simulink model "gm_testing"  (R2023a)
settings: Solver=VariableStepAuto  StartTime=0.0  StopTime=inf  RelTol=1e-3
libraries: commdigbbndpm3 x1, commrandsrc3 x1, simulink x1
settings Model: Creator=acer  LastModifiedBy=acer
settings OptimizationCC: BlockReduction=off  ConditionallyExecuteInputs=off
settings DebuggingCC: InheritedTsInSrcMsg=none

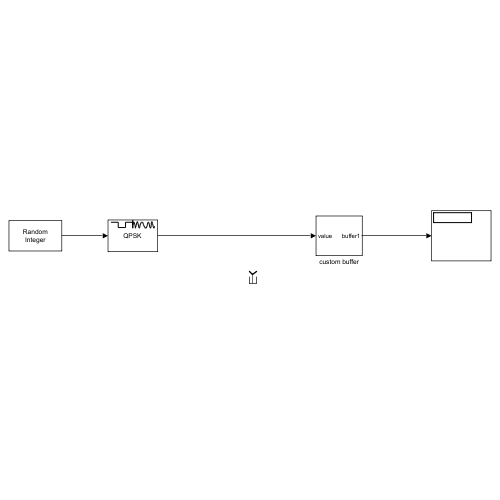
[thumbnail: Simulink's stored preview of the top-level diagram]
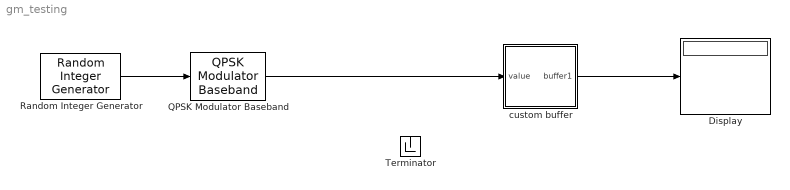
== system gm_testing ==
  Display : Display
  QPSK Modulator Baseband : commdigbbndpm3/QPSK Modulator Baseband  InType=Integer  Enc=Gray  Ph=pi/4  outDtype=Fixed-point  outWordLen=16  outUDDataType=sfix(16)  outFracLenMode=Best precision  outFracLen=15  outDataTypeStr=fixdt(1,16)  outLastDataTypeStr=fixdt(1,16)
      settings: LibrarySourceBlock=|
      | commhdldigbbndpm/QPSK
      | Modulator
      | Baseband
  Random Integer Generator : commrandsrc3/Random Integer Generator  SetSize=4  SeedSource=Auto  Seed=0  SampleTime=1  SamplesPerFrame=1  OutputDataType=uint8  SimulateUsing=Interpreted execution
  Terminator : Terminator
  custom buffer : Subsystem
  wires:
  QPSK Modulator Baseband/1 -> custom buffer/1(value)
  Random Integer Generator/1 -> QPSK Modulator Baseband/1
  custom buffer/1(buffer1) -> Display/1

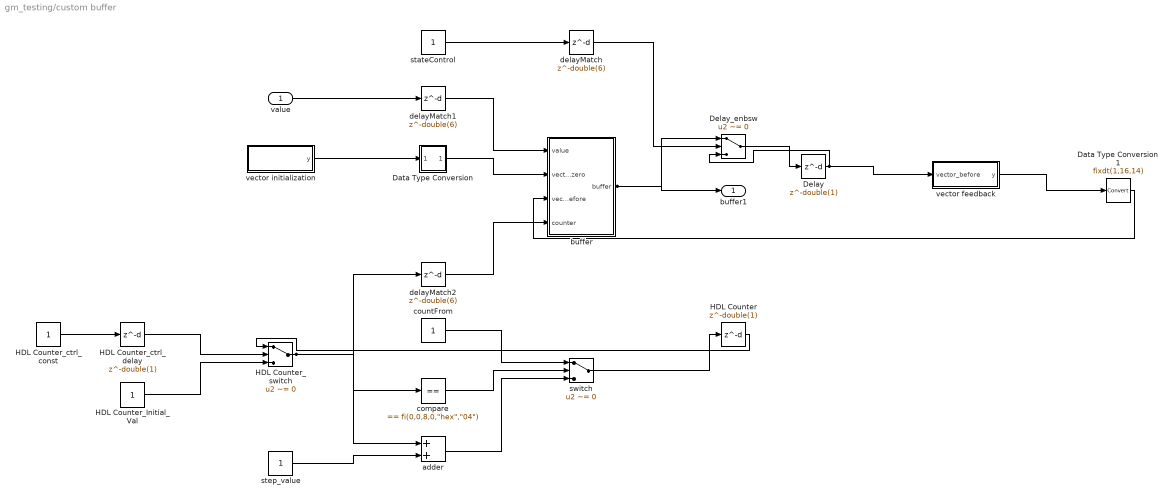
== system gm_testing/custom buffer ==
  value : Inport  OutDataTypeStr=fixdt(1, 16, 15)  PortDimensions=1  SampleTime=1
      settings: SignalType=complex
  Data Type Conversion : Subsystem
      mask Display: disp('NFP\nconv');
  Data Type Conversion1 : DataTypeConversion  OutDataTypeStr=fixdt(1,16,14)
  Delay : Delay  DelayLength=double(1)  InitialCondition=0  SampleTime=1
  Delay_enbsw : Switch  Criteria=u2 ~= 0  Threshold=double(0)  OutDataTypeStr=fixdt(1, 16, 14)  SampleTime=1  SaturateOnIntegerOverflow=off  InputSameDT=off
  HDL Counter : Delay  DelayLength=double(1)  InitialCondition=0  SampleTime=1
  HDL Counter_Initial_Val : Constant  OutDataTypeStr=uint8  SampleTime=1
  HDL Counter_ctrl_const : Constant  OutDataTypeStr=boolean  SampleTime=1
  HDL Counter_ctrl_delay : Delay  DelayLength=double(1)  InitialCondition=0  SampleTime=1
  HDL Counter_switch : Switch  Criteria=u2 ~= 0  Threshold=double(0)  OutDataTypeStr=uint8  SampleTime=1  SaturateOnIntegerOverflow=off  InputSameDT=off
  adder : Sum  AccumDataTypeStr=uint8  OutDataTypeStr=uint8  SampleTime=1
  buffer : Subsystem
  compare : simulink/Logic and Bit Operations/Compare To Constant  relop===  const="fi(0,0,8,0,\"hex\",\"04\")"  OutDataTypeStr=boolean
  countFrom : Constant  VectorParams1D=off  OutDataTypeStr=uint8  SampleTime=1
  delayMatch : Delay  DelayLength=double(6)  InitialCondition=0  SampleTime=1
  delayMatch1 : Delay  DelayLength=double(6)  InitialCondition=0  SampleTime=1
  delayMatch2 : Delay  DelayLength=double(6)  InitialCondition=0  SampleTime=1
  stateControl : Constant  OutDataTypeStr=boolean  SampleTime=1
  step_value : Constant  VectorParams1D=off  OutDataTypeStr=uint8  SampleTime=1
  switch : Switch  Criteria=u2 ~= 0  Threshold=double(0)  OutDataTypeStr=uint8  SampleTime=1  SaturateOnIntegerOverflow=off  InputSameDT=off
  vector feedback : Subsystem
  vector initialization : Subsystem
  buffer1 : Outport  SampleTime=1
  wires:
  delayMatch1/1 -> buffer/1(value)
  delayMatch2/1 -> buffer/4(counter)
  vector initialization/1(y) -> Data Type Conversion/1(In1)
  HDL Counter_switch/1 -> delayMatch2/1, compare/1, adder/1
  step_value/1 -> adder/2
  countFrom/1 -> switch/1
  HDL Counter_Initial_Val/1 -> HDL Counter_switch/3
  HDL Counter_ctrl_const/1 -> HDL Counter_ctrl_delay/1
  HDL Counter_ctrl_delay/1 -> HDL Counter_switch/2
  Data Type Conversion/1(Out1) -> buffer/2(vector_zero)
  delayMatch/1 -> Delay_enbsw/2
  stateControl/1 -> delayMatch/1
  value/1 -> delayMatch1/1
  buffer/1(buffer) -> buffer1/1, Delay_enbsw/1
  Delay/1 -> vector feedback/1(vector_before), Delay_enbsw/3
  Delay_enbsw/1 -> Delay/1
  vector feedback/1(y) -> Data Type Conversion1/1
  Data Type Conversion1/1 -> buffer/3(vector_before)
  HDL Counter/1 -> HDL Counter_switch/1
  switch/1 -> HDL Counter/1
  adder/1 -> switch/3
  compare/1 -> switch/2

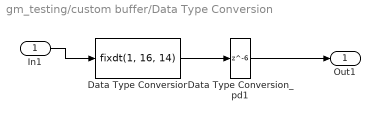
== system gm_testing/custom buffer/Data Type Conversion ==
  In1 : Inport
  Data Type Conversion : DataTypeConversion  OutDataTypeStr=fixdt(1, 16, 14)  SampleTime=1  SaturateOnIntegerOverflow=off  RndMeth=Floor
  Data Type Conversion_pd1 : Delay  DelayLength=6
  Out1 : Outport
  wires:
  In1/1 -> Data Type Conversion/1
  Data Type Conversion/1 -> Data Type Conversion_pd1/1
  Data Type Conversion_pd1/1 -> Out1/1

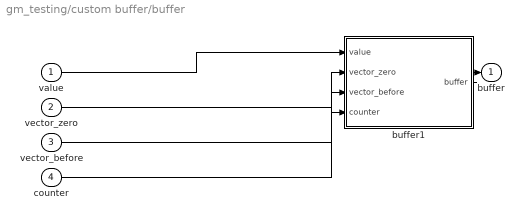
== system gm_testing/custom buffer/buffer ==
  value : Inport  OutDataTypeStr=fixdt(1, 16, 15)  PortDimensions=1  SampleTime=1
      settings: SignalType=complex
  vector_zero : Inport  Port=2  OutDataTypeStr=fixdt(1, 16, 14)  PortDimensions=[1 4]  SampleTime=1
      settings: SignalType=complex
  vector_before : Inport  Port=3  OutDataTypeStr=fixdt(1, 16, 14)  PortDimensions=[1 4]  SampleTime=1
      settings: SignalType=complex
  counter : Inport  Port=4  OutDataTypeStr=uint8  PortDimensions=1  SampleTime=1
  buffer1 : MATLAB Function  TreatAsAtomicUnit=on
  buffer : Outport  SampleTime=1
  wires:
  buffer1/1(buffer) -> buffer/1
  value/1 -> buffer1/1(value)
  vector_zero/1 -> buffer1/2(vector_zero)
  vector_before/1 -> buffer1/3(vector_before)
  counter/1 -> buffer1/4(counter)

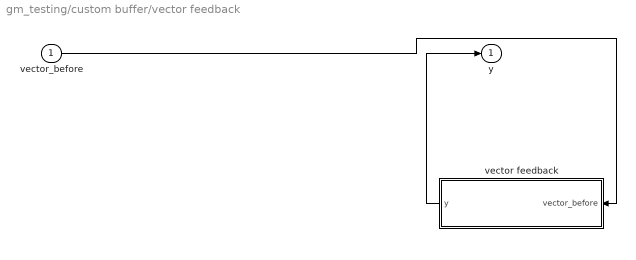
== system gm_testing/custom buffer/vector feedback ==
  vector_before : Inport  OutDataTypeStr=fixdt(1, 16, 14)  PortDimensions=[1 4]  SampleTime=1
      settings: SignalType=complex
  vector feedback : MATLAB Function  TreatAsAtomicUnit=on
  y : Outport  SampleTime=1  VectorParamsAs1DForOutWhenUnconnected=off
  wires:
  vector feedback/1(y) -> y/1
  vector_before/1 -> vector feedback/1(vector_before)

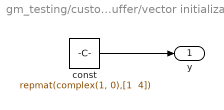
== system gm_testing/custom buffer/vector initialization ==
  const : Constant  Value="repmat(complex(1, 0),[1  4])"  VectorParams1D=off  OutDataTypeStr=double  SampleTime=1
  y : Outport  SampleTime=1  VectorParamsAs1DForOutWhenUnconnected=off
  wires:
  const/1 -> y/1

== matlab function gm_testing/custom buffer/buffer/buffer1 ==
  data: value input; vector_zero input; vector_before input; counter input; buffer output
function buffer = fcn(value, vector_zero, vector_before, counter)
%#codegen
if(counter == 0)
    buffer = vector_zero;
else
    buffer = vector_before;
end

buffer(counter) = value;

== matlab function gm_testing/custom buffer/vector feedback/vector feedback ==
  data: y output; vector_before input
function y = fcn(vector_before)
%#codegen

y = complex(vector_before);
